simulink model "vehicle_model_torque_distribution_equation"  (R2020b)
settings: Solver=VariableStepAuto  StartTime=0.0  StopTime=time  MaxStep=0.0001  RelTol=1e-12
values from neighbouring files (symbols this model uses):
  A = 2.71    [vehicle_parameters.m]
  chosen_input_t = t_sim5    [input_torque.m]
  chosen_input_T = input5    [input_torque.m]
  Cx = 0.31    [vehicle_parameters.m]
  f0 = 0.015    [vehicle_parameters.m]
  g = 9.81    [vehicle_parameters.m]
  hc = 0.5    [vehicle_parameters.m]
  It = 8    [vehicle_parameters.m]
  l = 2.73    [vehicle_parameters.m]
  lp = 1.2    [vehicle_parameters.m]
  lz = l - lp    (= 1.53)    [vehicle_parameters.m]
  m = 1700    [vehicle_parameters.m]
  mi = zeros(1,length(s))    [vehicle_parameters.m]
  rd = 0.3    [vehicle_parameters.m]
  ro = 1.2    [vehicle_parameters.m]
  s = -s_final:step:s_final    [vehicle_parameters.m]
  v0_sim = 16.67    [input_torque.m]
undefined symbols (not defined in the file or in its folder): mi_wet
settings Model: Creator=X  LastModifiedBy=X

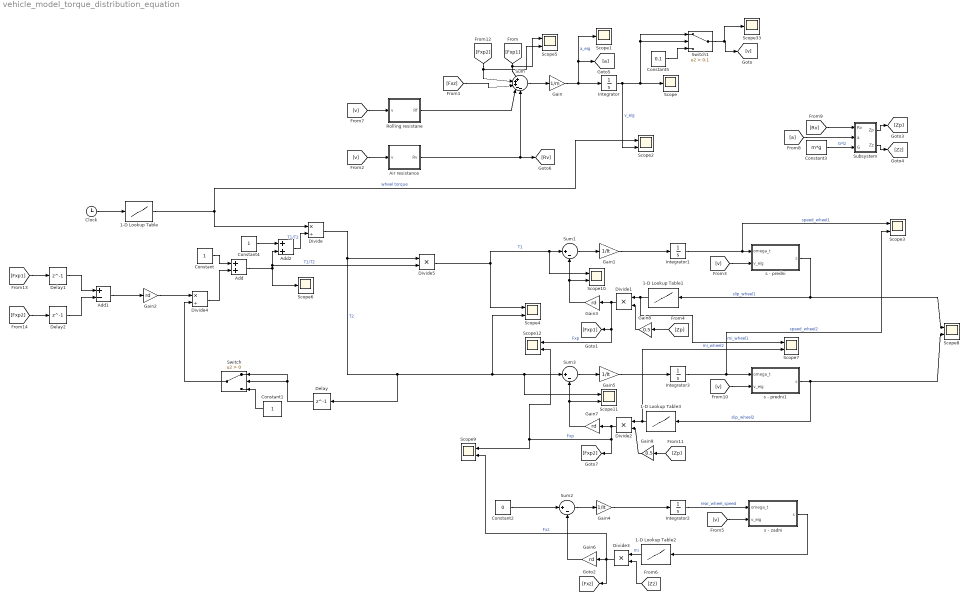
== system vehicle_model_torque_distribution_equation ==
  1-D Lookup Table : Lookup_n-D  NumberOfTableDimensions=1  BreakpointsForDimension1=chosen_input_t  Table=chosen_input_T  InternalRulePriority=Speed  RndMeth=Simplest  InputSameDT=on
  1-D Lookup Table1 : Lookup_n-D  NumberOfTableDimensions=1  BreakpointsForDimension1=s  Table=mi  InternalRulePriority=Speed  RndMeth=Simplest  InputSameDT=on
  1-D Lookup Table2 : Lookup_n-D  NumberOfTableDimensions=1  BreakpointsForDimension1=s  Table=mi  InternalRulePriority=Speed  RndMeth=Simplest  InputSameDT=on
  1-D Lookup Table3 : Lookup_n-D  NumberOfTableDimensions=1  BreakpointsForDimension1=s  Table=mi_wet  InternalRulePriority=Speed  RndMeth=Simplest  InputSameDT=on
  Add : Sum
  Add1 : Sum  Inputs=+-
  Add2 : Sum
  Air resistance : Subsystem
  Clock : Clock
  Constant : Constant
  Constant1 : Constant
  Constant2 : Constant  Value=0
  Constant3 : Constant  Value=m*g
  Constant4 : Constant
  Constant5 : Constant  Value=0.1
  Delay : Delay  DelayLength=1  InitialCondition=0
  Delay1 : Delay  DelayLength=1  InitialCondition=0
  Delay2 : Delay  DelayLength=1  InitialCondition=0
  Divide : Product  Inputs=*/
  Divide{1..3,5} (4 alike) : Product  Inputs=**
  Divide4 : Product  Inputs=*/
  Gain : Gain  Gain=1/m
  Gain1 : Gain  Gain=1/It
  Gain{2..3,6..7} (4 alike) : Gain  Gain=rd
  Gain4 : Gain  Gain=1/It
  Gain5 : Gain  Gain=1/It
  Gain8 : Gain  Gain=0.5
  Gain9 : Gain  Gain=0.5
  Integrator : Integrator  InitialCondition=v0_sim  ZeroCross=off
  Integrator1 : Integrator  InitialCondition=v0_sim/rd
  Integrator2 : Integrator  InitialCondition=v0_sim/rd
  Integrator3 : Integrator  InitialCondition=v0_sim/rd
  Rolling resistane : Subsystem
  Scope{,1,6,33} (4 alike) : Scope
  Scope{2..5,7..12} (10 alike) : Scope  NumInputPorts=2
  Subsystem : Subsystem
  Sum : Sum  Inputs=|+++--
  Sum1 : Sum  Inputs=|+-
  Sum2 : Sum  Inputs=|+-
  Sum3 : Sum  Inputs=|+-
  Switch : Switch  Criteria=u2 > Threshold
  Switch1 : Switch  Criteria=u2 > Threshold  Threshold=0.1
  s - predni : MATLAB Function  TreatAsAtomicUnit=on
  s - predni1 : MATLAB Function  TreatAsAtomicUnit=on
  s - zadni : MATLAB Function  TreatAsAtomicUnit=on
  wires:
  1-D Lookup Table2/1 -> Divide3/1  "mi"
  Constant5/1 -> Switch1/3
  Switch1/1 -> Scope33/1, [v]
  [Zp] -> Gain8/1
  Integrator/1 -> Switch1/1, Switch1/2, Scope/1, Scope2/2  "v_eig"
  1-D Lookup Table/1 -> Scope2/1, Divide/1  "wheel torque"
  Clock/1 -> 1-D Lookup Table/1
  Gain1/1 -> Integrator1/1
  [Fxz] -> Sum/3
  Gain6/1 -> Sum2/2
  Divide3/1 -> [Fxz], Scope9/2, Gain6/1  "Fxz"
  [v] -> s - zadni/2(v_eig)
  Constant2/1 -> Sum2/1
  [v] -> s - predni/2(v_eig)
  1-D Lookup Table1/1 -> Scope7/1, Divide1/1  "mi_wheel1"
  Sum2/1 -> Gain4/1
  [Zz] -> Divide3/2
  Integrator2/1 -> s - zadni/1(omega_t)  "rear_wheel_speed"
  Gain4/1 -> Integrator2/1
  Divide1/1 -> [Fxp1], Scope12/1, Gain3/1  "Fxp"
  Sum/1 -> Gain/1
  Sum1/1 -> Gain1/1
  s - zadni/1(s) -> 1-D Lookup Table2/1
  Gain3/1 -> Scope10/2, Sum1/2
  [Fxp1] -> Scope5/1, Sum/1
  Gain/1 -> Scope1/1, [a], Integrator/1  "a_eig"
  s - predni/1(s) -> Scope8/1, 1-D Lookup Table1/1  "slip_wheel1"
  [v] -> Rolling resistane/1(v)
  Rolling resistane/1(Rf) -> Sum/4
  Air resistance/1(Rv) -> Sum/5, [Rv]
  [v] -> Air resistance/1(v)
  Integrator1/1 -> Scope3/1, s - predni/1(omega_t)  "speed_wheel1"
  [Rv] -> Subsystem/1(Rv)
  [a] -> Subsystem/2(a)
  Constant3/1 -> Subsystem/3(G)  "G*lz"
  Subsystem/1(Zp) -> [Zp]
  Subsystem/2(Zz) -> [Zz]
  Integrator3/1 -> Scope3/2, s - predni1/1(omega_t)  "speed_wheel2"
  s - predni1/1(s) -> Scope8/2, 1-D Lookup Table3/1  "slip_wheel2"
  Gain7/1 -> Scope11/2, Sum3/2
  Sum3/1 -> Gain5/1
  Divide2/1 -> Gain7/1, [Fxp2], Scope9/1, Scope12/2  "Fxp"
  1-D Lookup Table3/1 -> Scope7/2, Divide2/1  "mi_wheel2"
  [v] -> s - predni1/2(v_eig)
  Gain5/1 -> Integrator3/1
  [Zp] -> Gain9/1
  [Fxp2] -> Scope5/2, Sum/2
  Constant/1 -> Add/1
  Divide/1 -> Delay/1, Scope4/2, Scope11/1, Sum3/1, Divide5/1  "T2"
  Add/1 -> Scope6/1, Add2/2, Divide5/2  "T1/T2"
  Divide4/1 -> Add/2
  [Fxp1] -> Delay1/1
  [Fxp2] -> Delay2/1
  Add1/1 -> Gain2/1
  Divide5/1 -> Scope10/1, Sum1/1, Scope4/1  "T1"
  Delay/1 -> Switch/1, Switch/2
  Constant1/1 -> Switch/3
  Switch/1 -> Divide4/2
  Constant4/1 -> Add2/1
  Add2/1 -> Divide/2  "T1/T2"
  Gain2/1 -> Divide4/1
  Gain8/1 -> Divide1/2
  Gain9/1 -> Divide2/2
  Delay2/1 -> Add1/2
  Delay1/1 -> Add1/1

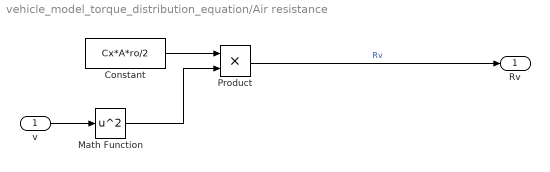
== system vehicle_model_torque_distribution_equation/Air resistance ==
  v : Inport
  Constant : Constant  Value=Cx*A*ro/2
  Math Function : Math  Operator=square  SaturateOnIntegerOverflow=on
  Product : Product
  Rv : Outport
  wires:
  Constant/1 -> Product/1
  Math Function/1 -> Product/2
  v/1 -> Math Function/1
  Product/1 -> Rv/1  "Rv"

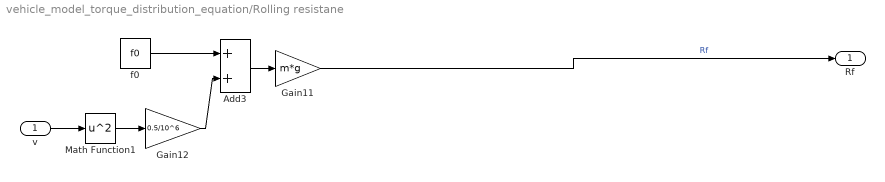
== system vehicle_model_torque_distribution_equation/Rolling resistane ==
  v : Inport
  Add3 : Sum
  Gain11 : Gain  Gain=m*g
  Gain12 : Gain  Gain=0.5/10^6
  Math Function1 : Math  Operator=square  SaturateOnIntegerOverflow=on
  f0 : Constant  Value=f0
  Rf : Outport
  wires:
  Math Function1/1 -> Gain12/1
  f0/1 -> Add3/1
  Add3/1 -> Gain11/1
  Gain12/1 -> Add3/2
  v/1 -> Math Function1/1
  Gain11/1 -> Rf/1  "Rf"

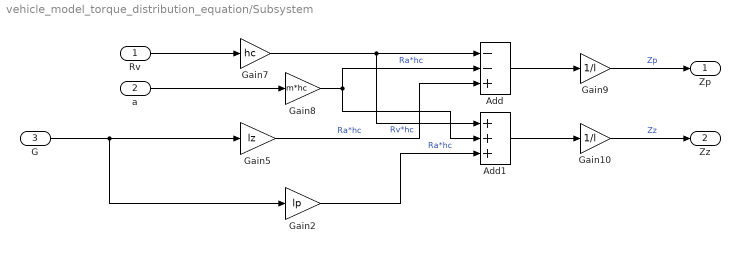
== system vehicle_model_torque_distribution_equation/Subsystem ==
  Rv : Inport
  a : Inport  Port=2
  G : Inport  Port=3
  Add : Sum  Inputs=--+
  Add1 : Sum  Inputs=+++
  Gain10 : Gain  Gain=1/l
  Gain2 : Gain  Gain=lp
  Gain5 : Gain  Gain=lz
  Gain7 : Gain  Gain=hc
  Gain8 : Gain  Gain=m*hc
  Gain9 : Gain  Gain=1/l
  Zp : Outport
  Zz : Outport  Port=2
  wires:
  G/1 -> Gain2/1, Gain5/1
  Gain10/1 -> Zz/1  "Zz"
  Gain8/1 -> Add/2, Add1/2  "Ra*hc"
  Add/1 -> Gain9/1
  Gain7/1 -> Add1/1, Add/1  "Rv*hc"
  Gain2/1 -> Add1/3  "Ra*hc"
  Add1/1 -> Gain10/1
  Gain5/1 -> Add/3  "Ra*hc"
  Rv/1 -> Gain7/1
  Gain9/1 -> Zp/1  "Zp"
  a/1 -> Gain8/1

== matlab function vehicle_model_torque_distribution_equation/s - predni ==
  data: omega_t input; s output; v_eig input
function s = fcn(omega_t, v_eig)
rd = 0.3;
if omega_t*rd >= v_eig
    s = (omega_t*rd - v_eig)/(omega_t*rd);
else
    s = (omega_t*rd - v_eig)/v_eig;
end

== matlab function vehicle_model_torque_distribution_equation/s - predni1 ==
  data: omega_t input; s output; v_eig input
function s = fcn(omega_t, v_eig)
rd = 0.3;
if omega_t*rd >= v_eig
    s = (omega_t*rd - v_eig)/(omega_t*rd);
else
    s = (omega_t*rd - v_eig)/v_eig;
end

== matlab function vehicle_model_torque_distribution_equation/s - zadni ==
  data: omega_t input; s output; v_eig input
function s = fcn(omega_t, v_eig)
rd = 0.3;
if omega_t*rd >= v_eig
    s = (omega_t*rd - v_eig)/(omega_t*rd);
else
    s = (omega_t*rd - v_eig)/v_eig;
end
